simulink model "AproxDiscreteComparison"  (R2021a)
settings: Solver=FixedStepAuto  StartTime=0.0  StopTime=SimTime  FixedStep=1e-3  RelTol=1e-3
values from neighbouring files (symbols this model uses):
  Tq = 1e-2    (= 0.01)    [ComparisonDiscresization.m]    (also in DigitalPIDRunner.m = 0.001; NNTrainingSet.m = 0.1; reference.mat = 0.1)
settings Model: Creator=akangmufti  LastModifiedBy=akangmufti

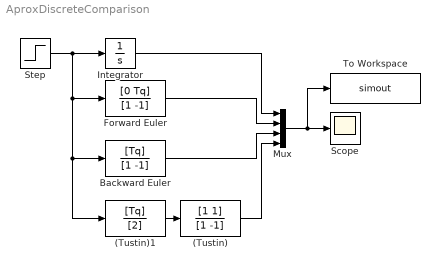
== system AproxDiscreteComparison ==
  (Tustin) : DiscreteFilter  Numerator=[1 1]  Denominator=[1 -1]  SampleTime=Tq
  (Tustin)1 : DiscreteFilter  Numerator=[Tq]  Denominator=[2]  SampleTime=Tq
  Backward Euler : DiscreteFilter  Numerator=[Tq]  Denominator=[1 -1]  SampleTime=Tq
  Forward Euler : DiscreteFilter  Numerator=[0 Tq]  Denominator=[1 -1]  SampleTime=Tq
  Integrator : Integrator
  Mux : Mux
  Scope : Scope
  Step : Step  Time=Tq  SampleTime=0
  To Workspace : ToWorkspace  VariableName=simout  SampleTime=1e-3
  wires:
  (Tustin)1/1 -> (Tustin)/1
  Step/1 -> (Tustin)1/1, Backward Euler/1, Forward Euler/1, Integrator/1
  Mux/1 -> To Workspace/1, Scope/1
  Integrator/1 -> Mux/1
  Forward Euler/1 -> Mux/2
  Backward Euler/1 -> Mux/3
  (Tustin)/1 -> Mux/4
